simulink model "LEO_MPCACC_VLV1"  (Simulink 8.2)
settings: Solver=ode45  StartTime=0.0  StopTime=40  RelTol=1e-3
libraries: Solver_SF x2
settings Model: Creator=admin  LastModifiedBy=leoking99
settings DataIOCC: SignalLoggingSaveFormat=Dataset
settings OptimizationCC: ExpressionDepthLimit=128
settings DebuggingCC: FcnCallInpInsideContextMsg=EnableAllAsError  StateNameClashWarn=none
settings GRTTargetCC: CombineOutputUpdateFcns=on  GRTInterface=off

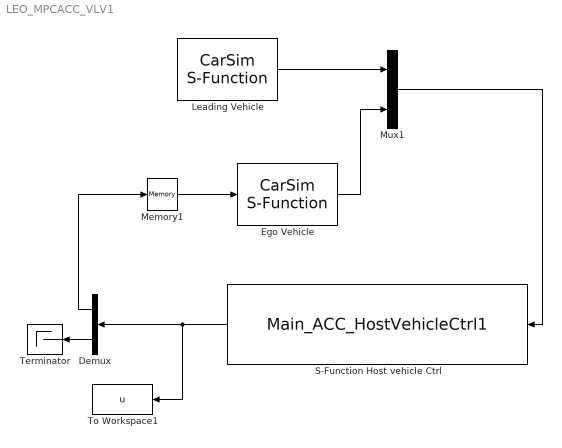
== system LEO_MPCACC_VLV1 ==
  Demux : Demux  Outputs=[3 6]
  Ego Vehicle : Solver_SF/CarSim S-Function  Priority=1  VehicleCode=i_i2_64  SIMFILE=LEO_MPC_ACC_ExtSen_Car2.sim
  Leading Vehicle : Solver_SF/CarSim S-Function  Priority=1  VehicleCode=i_i  SIMFILE=LEO_MPC_ACC_ExtSen_Car1.sim
  Memory1 : Memory
  Mux1 : Mux  Inputs=2
  S-Function Host vehicle Ctrl : S-Function  FunctionName=Main_ACC_HostVehicleCtrl1  EnableBusSupport=off
  Terminator : Terminator
  To Workspace1 : ToWorkspace  VariableName=u  SampleTime=-1  SaveFormat=Structure
  wires:
  S-Function Host vehicle Ctrl/1 -> To Workspace1/1, Demux/1
  Demux/1 -> Memory1/1
  Demux/2 -> Terminator/1
  Memory1/1 -> Ego Vehicle/1
  Ego Vehicle/1 -> Mux1/2
  Mux1/1 -> S-Function Host vehicle Ctrl/1
  Leading Vehicle/1 -> Mux1/1
